simulink model "copysprzezenie_od_stanu2"  (R2017b)
settings: Solver=VariableStepAuto  StartTime=0.0  StopTime=10  RelTol=1e-3
values from neighbouring files (symbols this model uses):
  A2 = [3.22791678547  1  0; -1.44925930399  0  1; 0.17377394345  0  0]    [matlab.mat]
  B2 = [0.260707487539 -0.289205764977 0.0761198486843]    [matlab.mat]
  K = [11.2993624638 4.84519726655 2.40866701447]    [matlab.mat]
  Tp = 0.25    [matlab.mat]
  x_start = [3 -2 1]    [matlab.mat]
settings Model: Creator=gulin  LastModifiedBy=gulin

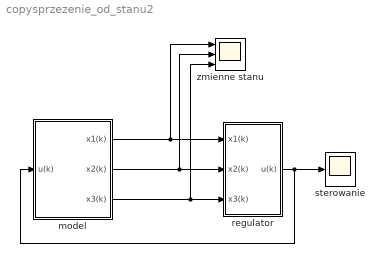
== system copysprzezenie_od_stanu2 ==
  model : Subsystem
  regulator : Subsystem
  sterowanie : Scope
  "zmienne stanu " : Scope  NumInputPorts=3
  wires:
  model/1("x1(k) ") -> "zmienne stanu "/1, regulator/1(x1(k))
  model/2(x2(k)) -> "zmienne stanu "/2, regulator/2(x2(k))
  model/3(x3(k)) -> "zmienne stanu "/3, regulator/3(x3(k))
  regulator/1(u(k)) -> sterowanie/1, model/1("u(k) ")

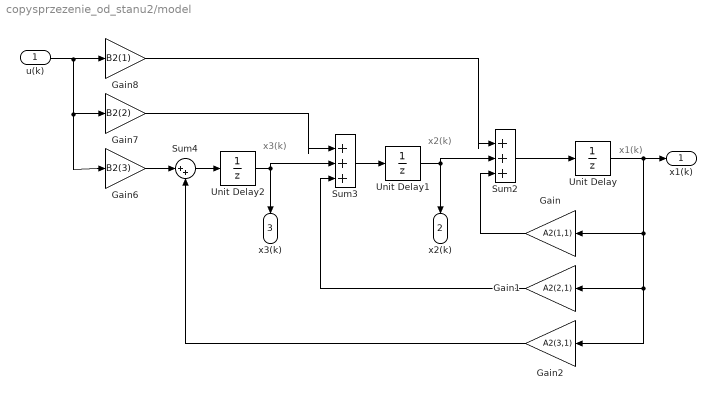
== system copysprzezenie_od_stanu2/model ==
  note: x1(k)
  note: x3(k)
  note: x2(k)
  "u(k) " : Inport
  Gain : Gain  Gain=A2(1,1)
  Gain1 : Gain  Gain=A2(2,1)
  Gain2 : Gain  Gain=A2(3,1)
  Gain6 : Gain  Gain=B2(3)
  Gain7 : Gain  Gain=B2(2)
  Gain8 : Gain  Gain=B2(1)
  Sum2 : Sum  Inputs=|+++
  Sum3 : Sum  Inputs=|+++
  Sum4 : Sum  Inputs=|++
  Unit Delay : UnitDelay  InitialCondition=x_start(1)  SampleTime=Tp
  Unit Delay1 : UnitDelay  InitialCondition=x_start(2)  SampleTime=Tp
  Unit Delay2 : UnitDelay  InitialCondition=x_start(3)  SampleTime=Tp
  "x1(k) " : Outport
  x2(k) : Outport  Port=2
  x3(k) : Outport  Port=3
  wires:
  Gain1/1 -> Sum3/3
  Gain2/1 -> Sum4/2
  Sum2/1 -> Unit Delay/1
  Sum4/1 -> Unit Delay2/1
  Unit Delay2/1 -> Sum3/2, x3(k)/1
  Gain7/1 -> Sum3/1
  Sum3/1 -> Unit Delay1/1
  Gain/1 -> Sum2/3
  Unit Delay/1 -> Gain2/1, Gain1/1, Gain/1, "x1(k) "/1
  Gain6/1 -> Sum4/1
  Gain8/1 -> Sum2/1
  "u(k) "/1 -> Gain7/1, Gain6/1, Gain8/1
  Unit Delay1/1 -> Sum2/2, x2(k)/1

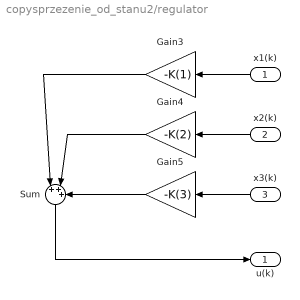
== system copysprzezenie_od_stanu2/regulator ==
  x1(k) : Inport
  x2(k) : Inport  Port=2
  x3(k) : Inport  Port=3
  Gain3 : Gain  Gain=-K(1)
  Gain4 : Gain  Gain=-K(2)
  Gain5 : Gain  Gain=-K(3)
  Sum : Sum  Inputs=|+++
  u(k) : Outport
  wires:
  Gain4/1 -> Sum/2
  Gain3/1 -> Sum/1
  Sum/1 -> u(k)/1
  Gain5/1 -> Sum/3
  x2(k)/1 -> Gain4/1
  x1(k)/1 -> Gain3/1
  x3(k)/1 -> Gain5/1
